simulink model "e8_t2"  (R2025b)
settings: Solver=VariableStepAuto  StartTime=0.0  StopTime=1  RelTol=1e-3
PostLoadFcn:
  | load('acceleration.mat');
settings Model: LastModifiedBy=Hamidur

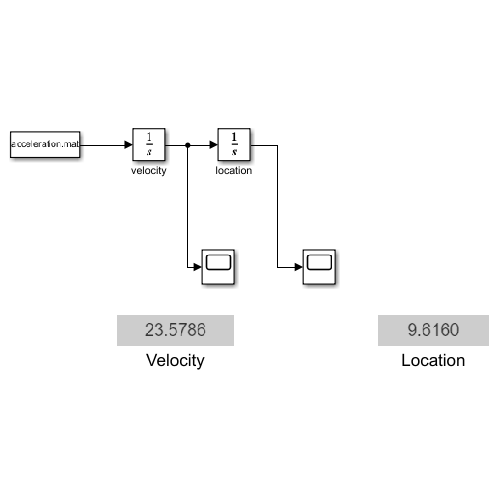
[thumbnail: Simulink's stored preview of the top-level diagram]
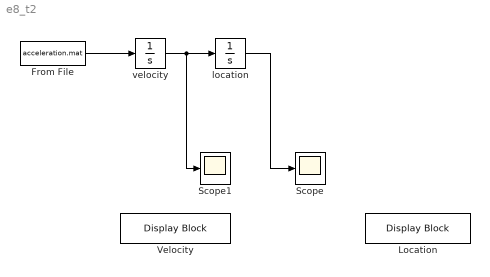
== system e8_t2 ==
  From File : FromFile  FileName=acceleration.mat  SampleTime=0
  Location : DisplayBlock  LabelPosition=Hide  Transparency=1  GridColor=[0.502, 0.502, 0.502]
  Scope : Scope
  Scope1 : Scope
  Velocity : DisplayBlock  LabelPosition=Hide  Transparency=1  GridColor=[0.502, 0.502, 0.502]
  location : Integrator
  velocity : Integrator
  wires:
  velocity/1 -> Scope1/1, location/1
  location/1 -> Scope/1
  From File/1 -> velocity/1
